simulink model "PSK"  (R2014a)
settings: Solver=ode45  StartTime=0.0  StopTime=10.0  RelTol=1e-3
settings Model: Creator=admin  LastModifiedBy=admin

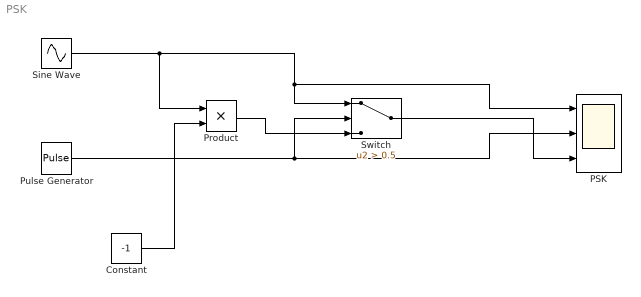
== system PSK ==
  Constant : Constant  Value=-1
  PSK : Scope  NumInputPorts=3
      settings: YMin=-5~-5~-5  YMax=5~5~5
  Product : Product
  Pulse Generator : DiscretePulseGenerator  PulseType=Time based  Amplitude=3  PulseWidth=50
  Sine Wave : Sin  Amplitude=3  Frequency=2*pi*2  SampleTime=0.01
  Switch : Switch  Criteria=u2 > Threshold  Threshold=0.5
  wires:
  Sine Wave/1 -> Product/1, PSK/1, Switch/1
  Pulse Generator/1 -> PSK/2, Switch/2
  Constant/1 -> Product/2
  Product/1 -> Switch/3
  Switch/1 -> PSK/3
